simulink model "averagebuck"  (R2018b)
settings: Solver=VariableStepAuto  StartTime=0.0  StopTime=10.0  RelTol=1e-3
libraries: simulink x1
settings Model: Creator=Soto Porras  LastModifiedBy=Soto Porras

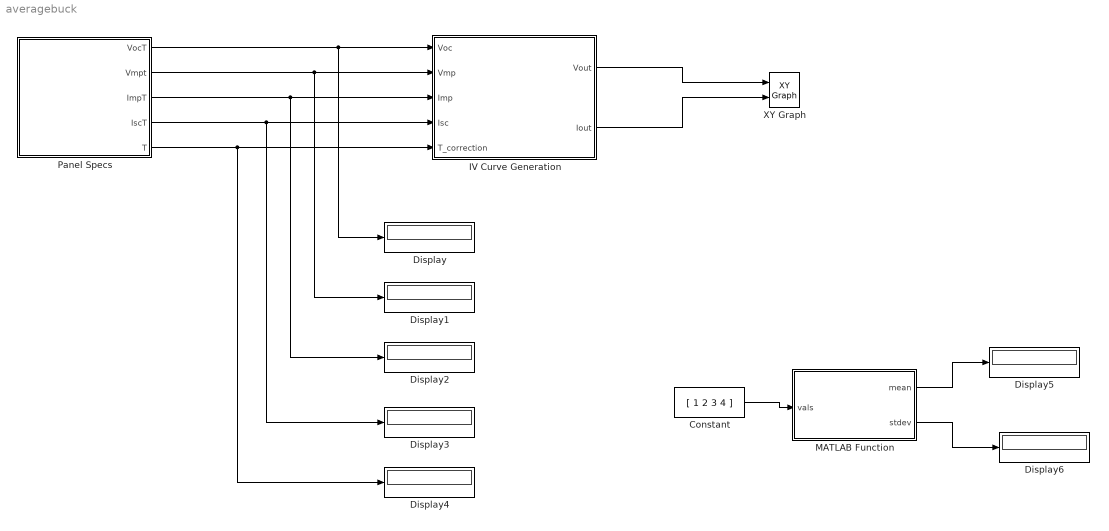
== system averagebuck ==
  Constant : Constant  Value=[ 1 2 3 4 ]
  Display{,1..6} (7 alike) : Display
  IV Curve Generation : Subsystem  mask(Panel I-V Curve Calculation){ValueVocComp=0.0062, ValueVmpComp=0.0067}
      mask prompts: ValueVocComp "Voc Temperature Correction (V)"; ValueVmpComp "Vmp Temperature Correction (V)"
      mask help:
      | This module calculates the panel IV curve using the next panel parameters:
      | 1. Voc
      | 2. Vmp
      | 3. Imp
      | 4. Isc
      |
      | It applies:
      | 1. Correction to current parameters (Isc and Imp) using a pseudo cosine that varies depending on the angle of the perpendicular CubeSat face and the sun's incident radiation.
      | 2. Correction to voltage parameters (Voc and Vmp) using the panel datasheet voltage losses, given in V by the user.
      mask TypeOptions ValueVocComp: Voc_comp/Value
      mask TypeOptions ValueVmpComp: Vmp_comp/Value
      mask Display: image('IV_curve.png');
  MATLAB Function : MATLAB Function  TreatAsAtomicUnit=on
  Panel Specs : Subsystem  mask(Solar Panel Specifications){Voc=2.690, Vmp=2.409, Imp=0.5029, Isc=0.5196, Temp=28, SerialGain=2, ParallelGain=3}
      mask prompts: Temp "T°"; SerialGain "Serial"; ParallelGain "Parallel"
      mask help: Inputs solar panel electrical specifications, temperature and array distribution.
      mask TypeOptions Voc: Voc/Value
      mask TypeOptions Vmp: Vmp/Value
      mask TypeOptions Imp: Imp/Value
      mask TypeOptions Isc: Isc/Value
      mask TypeOptions Temp: T°/Value
      mask TypeOptions SerialGain: Gain/Gain | Gain1/Gain
      mask TypeOptions ParallelGain: Gain2/Gain | Gain3/Gain
      mask DialogControl Container3 Prompt: Panel Array
      mask Display: image('solar_panel.png');
  XY Graph : simulink/Sinks/XY Graph  xmin=-1  xmax=1  ymin=-1  ymax=1  st=-1
  wires:
  Panel Specs/1(VocT) -> Display/1, IV Curve Generation/1(Voc)
  Panel Specs/2(Vmpt) -> Display1/1, IV Curve Generation/2(Vmp)
  Panel Specs/3(ImpT) -> Display2/1, IV Curve Generation/3(Imp)
  Panel Specs/4(IscT) -> Display3/1, IV Curve Generation/4(Isc)
  Panel Specs/5(T) -> Display4/1, IV Curve Generation/5(T_correction)
  Constant/1 -> MATLAB Function/1(vals)
  MATLAB Function/2(stdev) -> Display6/1
  MATLAB Function/1(mean) -> Display5/1
  IV Curve Generation/1(Vout) -> XY Graph/1
  IV Curve Generation/2(Iout) -> XY Graph/2

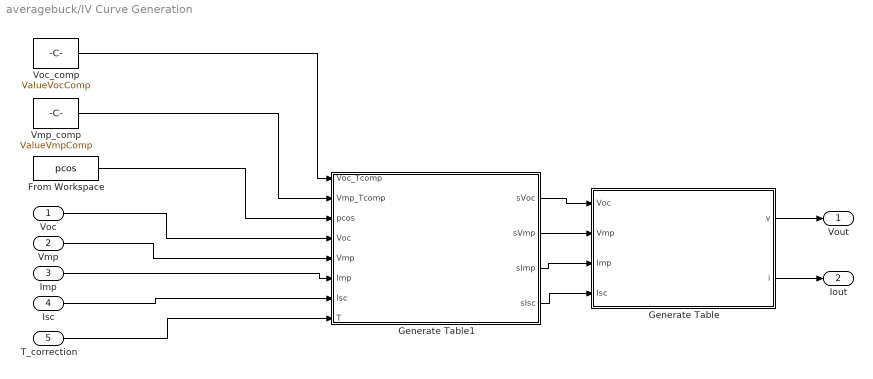
== system averagebuck/IV Curve Generation ==
  Voc : Inport
  Vmp : Inport  Port=2
  Imp : Inport  Port=3
  Isc : Inport  Port=4
  T_correction : Inport  Port=5
  From Workspace : FromWorkspace  VariableName=pcos  SampleTime=0
  Generate Table : MATLAB Function  TreatAsAtomicUnit=on
  Generate Table1 : MATLAB Function  TreatAsAtomicUnit=on
  Vmp_comp : Constant  Value=ValueVmpComp
  Voc_comp : Constant  Value=ValueVocComp
  Vout : Outport
  Iout : Outport  Port=2
  wires:
  Isc/1 -> Generate Table1/7(Isc)
  Generate Table1/4(sIsc) -> Generate Table/4(Isc)
  Voc_comp/1 -> Generate Table1/1(Voc_Tcomp)
  Generate Table/1(v) -> Vout/1
  T_correction/1 -> Generate Table1/8(T)
  Generate Table1/2(sVmp) -> Generate Table/2(Vmp)
  Voc/1 -> Generate Table1/4(Voc)
  From Workspace/1 -> Generate Table1/3(pcos)
  Generate Table1/3(sImp) -> Generate Table/3(Imp)
  Imp/1 -> Generate Table1/6(Imp)
  Generate Table1/1(sVoc) -> Generate Table/1(Voc)
  Vmp/1 -> Generate Table1/5(Vmp)
  Generate Table/2(i) -> Iout/1
  Vmp_comp/1 -> Generate Table1/2(Vmp_Tcomp)

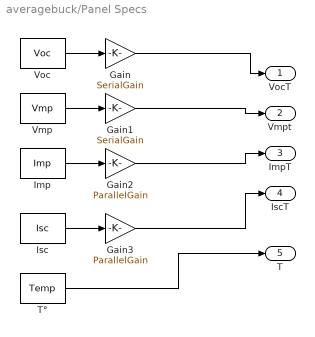
== system averagebuck/Panel Specs ==
  Gain : Gain  Gain=SerialGain
  Gain1 : Gain  Gain=SerialGain
  Gain2 : Gain  Gain=ParallelGain
  Gain3 : Gain  Gain=ParallelGain
  Imp : Constant  Value=Imp
  Isc : Constant  Value=Isc
  T° : Constant  Value=Temp
  Vmp : Constant  Value=Vmp
  Voc : Constant  Value=Voc
  VocT : Outport
  Vmpt : Outport  Port=2
  ImpT : Outport  Port=3
  IscT : Outport  Port=4
  T : Outport  Port=5
  wires:
  Isc/1 -> Gain3/1
  Vmp/1 -> Gain1/1
  Gain/1 -> VocT/1
  Imp/1 -> Gain2/1
  Gain2/1 -> ImpT/1
  Gain3/1 -> IscT/1
  Voc/1 -> Gain/1
  Gain1/1 -> Vmpt/1
  T°/1 -> T/1

== matlab function averagebuck/MATLAB Function ==
  data: vals input; mean output; stdev output
function [mean,stdev] = stats(vals)
    % Calculates a statistical mean and a standard
    % deviation for the values in vals.

    len = length(vals);
    mean = avg(vals,len);
    stdev = sqrt(sum(((vals-avg(vals,len)).^2))/len);
    plot(vals,'-+');
    
end

== matlab function averagebuck/IV Curve Generation/Generate Table ==
  data: Voc input; Vmp input; Imp input; Isc input; v output; i output
function [v,i] = generate_table(Voc, Vmp, Imp, Isc)
Rs = ( Voc - Vmp ) / Imp;
a = ( Vmp * ( 1 + ( Rs*Isc ) / Voc ) + Rs*( Imp - Isc ) ) / Voc;
N = log( 2 - 2^a) / log ( Imp / Isc );
i=zeros(1024,1);
v=zeros(1024,1);
for x = 1:1024
    I = (x * Isc) / 1023.0;
    V = Voc * log( 2 - ( ( I / Isc ) ^ N ) );
    V = V / log( 2 );
    V = V - Rs * ( I - Isc );
    V = V / ( 1 + ( ( Rs * Isc) / Voc) );
    P = V * I;
    v(x) = V;
    i(x) = I;
end
v = flip(v);
i = flip(i);

== matlab function averagebuck/IV Curve Generation/Generate Table1 ==
  data: Voc_Tcomp input; Vmp_Tcomp input; pcos input; Voc input; Vmp input; Imp input; Isc input; sVoc output; sVmp output; sImp output; sIsc output; T input
function [sVoc, sVmp, sImp, sIsc] = scalevars(Voc_Tcomp, Vmp_Tcomp, pcos, Voc, Vmp, Imp, Isc, T)
sVoc = Voc-(T*Voc_Tcomp);
sVmp = Vmp-(T*Vmp_Tcomp);
sImp = pcos * Imp;
sIsc = pcos * Isc;
